simulink model "attitude_determination"  (R2024b)
settings: Solver=VariableStepAuto  StartTime=0.0  StopTime=inf  RelTol=1e-3
libraries: simulink x1
settings Model: Creator=boude  LastModifiedBy=boude

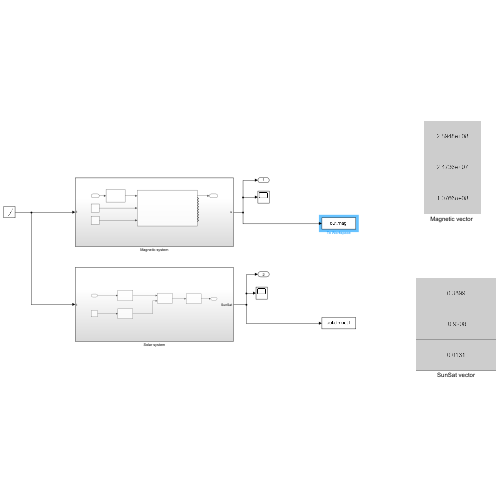
[thumbnail: Simulink's stored preview of the top-level diagram]
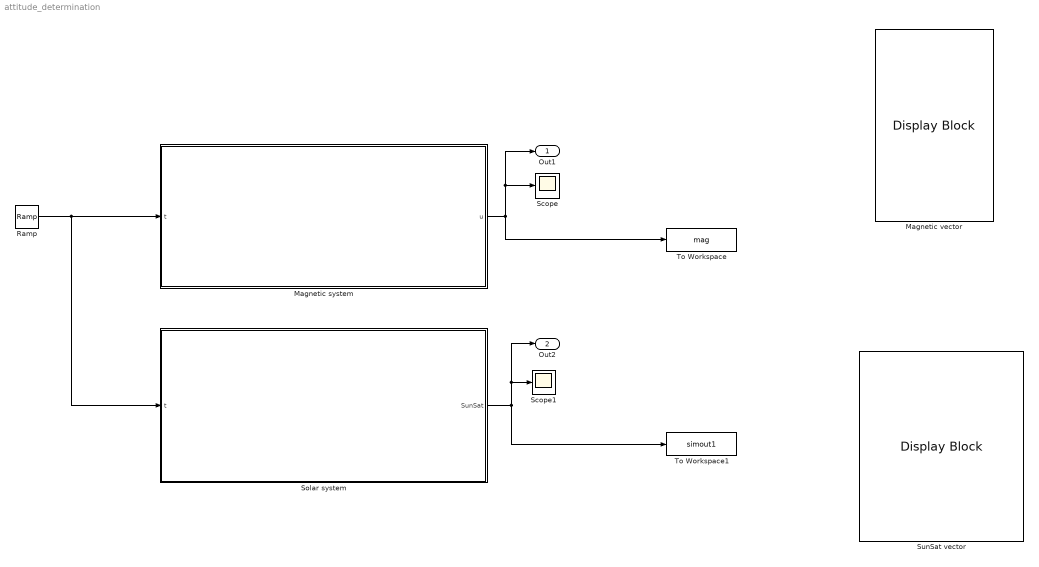
== system attitude_determination ==
  Magnetic system : Subsystem
  "Magnetic vector " : DisplayBlock  LabelPosition=Hide  Transparency=1  Layout=Fill available space
  Ramp : simulink/Sources/Ramp  slope=1  start=1  InitialOutput=1
  Scope : Scope
  Scope1 : Scope
  Solar system : Subsystem
  SunSat vector : DisplayBlock  LabelPosition=Hide  Transparency=1
  To Workspace : ToWorkspace  VariableName=mag  SampleTime=-1
      settings: Save2DSignal=2-D array (concatenate along first dimension)
  To Workspace1 : ToWorkspace  VariableName=simout1  SaveFormat=Timeseries  SampleTime=-1
  Out1 : Outport
  Out2 : Outport  Port=2
  wires:
  Ramp/1 -> Solar system/1(t), Magnetic system/1(t)
  Magnetic system/1(u) -> To Workspace/1, Out1/1, Scope/1
  Solar system/1(SunSat) -> To Workspace1/1, Out2/1, Scope1/1

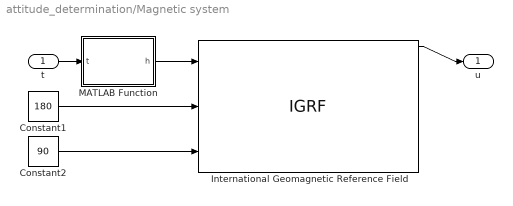
== system attitude_determination/Magnetic system ==
  t : Inport
  Constant1 : Constant  Value=180
  Constant2 : Constant  Value=90
  International Geomagnetic Reference Field : IGRF  units=English  time_in=off  month=December  day=6  year=2003
      settings: AttributesFormatString=%<generation>
  MATLAB Function : MATLAB Function  TreatAsAtomicUnit=on
  u : Outport
  wires:
  International Geomagnetic Reference Field/1 -> u/1
  Constant2/1 -> International Geomagnetic Reference Field/3
  Constant1/1 -> International Geomagnetic Reference Field/2
  MATLAB Function/1(h) -> International Geomagnetic Reference Field/1
  t/1 -> MATLAB Function/1(t)

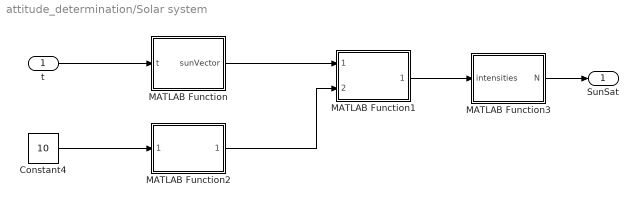
== system attitude_determination/Solar system ==
  t : Inport
  Constant4 : Constant  Value=10
  MATLAB Function : MATLAB Function  TreatAsAtomicUnit=on
  MATLAB Function1 : MATLAB Function  TreatAsAtomicUnit=on
  MATLAB Function2 : MATLAB Function  TreatAsAtomicUnit=on
  MATLAB Function3 : MATLAB Function  TreatAsAtomicUnit=on
  SunSat : Outport
  wires:
  Constant4/1 -> MATLAB Function2/1(omega)
  MATLAB Function/1(sunVector) -> MATLAB Function1/1(sunVec)
  MATLAB Function2/1(R_cubesat) -> MATLAB Function1/2(R_cubesat)
  t/1 -> MATLAB Function/1(t)
  MATLAB Function1/1(intensities) -> MATLAB Function3/1(intensities)
  MATLAB Function3/1(N) -> SunSat/1

== matlab function attitude_determination/Solar system/MATLAB Function ==
  data: t input; sunVector output
function sunVector  = sunPositionSimple(t)
% sunPositionSimple : calcul approximatif du vecteur unitaire pointant vers le Soleil
% Inputs:
%   - dayOfYear : jour de l'année (1 à 365)
%   - timeUTC : heure en décimal UTC (ex: 13.5 = 13h30 UTC)
% Output:
%   - sunVector : vecteur 3D unitaire [x;y;z] pointant vers le soleil en coordonnées ENU (Est-Nord-Haut)
    dayOfYear = floor(t / 86400) + 1;
    timeUTC = mod(t, 86400) / 3600;  % heure en décimal

    % Constantes
    lat = 48.8566;    % latitude Paris (°)
    lon = 2.3522;     % longitude Paris (°)
    
    % Calcul de l'angle horaire solaire (en degrés)
    % On suppose que midi solaire correspond à 12h heure locale
    % Correction décalage longitude vers UTC
    localTime = timeUTC + lon/15; % Convertit UTC en heure solaire approximative locale
    
    % Angle horaire solaire (omega) en degrés, midi solaire = 0°, matin négatif, après-midi positif
    omega = 15 * (localTime - 12);
    
    % Déclinaison solaire approximative (en degrés)
    % Approximation simple en fonction du jour de l'année (formule trigonométrique)
    declin = 23.44 * sind(360 * (284 + dayOfYear) / 365);
    
    % Calcul de l'angle zénithal solaire (theta_sun)
    cos_theta = sind(lat) * sind(declin) + cosd(lat) * cosd(declin) * cosd(omega);
    theta_sun = acosd(cos_theta);  % en degrés
    
    % Calcul de l'azimut solaire (phi_sun) approximatif (degrés, depuis le sud, vers l'ouest)
    sin_phi = -(cosd(declin) * sind(omega)) / sind(theta_sun);
    cos_phi = (sind(declin) - sind(lat) * cosd(theta_sun)) / (cosd(lat) * sind(theta_sun));
    phi_sun = atan2d(sin_phi, cos_phi);
    
    % Passage à un vecteur unitaire (système de coordonnées ENU)
    % x = Est, y = Nord, z = Haut
    % Azimut depuis le sud vers l'ouest → on recentre vers Est = 0°, Nord = 90°
    azimuth = mod(180 - phi_sun, 360); % azimut en degrés, 0 = Est, 90 = Nord
    
    % Convertir en radians
    zenith_rad = deg2rad(theta_sun);
    azimuth_rad = deg2rad(azimuth);
    
    % Composantes cartésiennes
    x = sin(zenith_rad) * cos(azimuth_rad);
    y = sin(zenith_rad) * sin(azimuth_rad);
    z = cos(zenith_rad);
    
    sunVector = [x; y; z];

    if theta_sun > 90
        sunVector = [0; 0; 0];
    end
    
end

== matlab function attitude_determination/Solar system/MATLAB Function2 ==
  data: omega input; R_cubesat output
function R_cubesat = fcn(omega)
t = 60;
theta = deg2rad(omega * t); % omega in deg/s, t in seconds
R_cubesat = [cos(theta), -sin(theta), 0;
     sin(theta),  cos(theta), 0;
     0,           0,          1];

== matlab function attitude_determination/Magnetic system/MATLAB Function ==
  data: h output; t input
function h = altitudeVariation(t)
% altitudeVariation : donne l'altitude en fonction du temps t (en secondes)
% h(t) = 500 + 100 * sin(2π * t / 600)

    h = 500 + 100 * sin(2 * pi * t / 600);
end

== matlab function attitude_determination/Solar system/MATLAB Function3 ==
  data: intensities input; N output
function N = sunSatelliteVector(intensities)
% sunSatelliteVector : calcule le vecteur Soleil-Satellite à partir des intensités mesurées
% Input:
%   - intensities : [6x1] vecteur contenant l’intensité sur chaque panneau solaire
% Output:
%   - N : [3x1] vecteur unitaire directionnel Soleil-Satellite

    % Normales des 6 faces du CubeSat (X+, X-, Y+, Y-, Z+, Z-)
    normals = [ 1  0  0;   % Face X+
               -1  0  0;   % Face X-
                0  1  0;   % Face Y+
                0 -1  0;   % Face Y-
                0  0  1;   % Face Z+
                0  0 -1];  % Face Z-

    % Numérateur : somme pondérée des normales
    numerator = zeros(1,3);
    for i = 1:6
        numerator = numerator + intensities(i) * normals(i,:);
    end

    % Dénominateur : somme des intensités
    denominator = sum(intensities);

    % Si toutes les intensités sont nulles → soleil non visible
    if denominator < 1e-3  % seuil de sécurité
        N = [0; 0; 0];  % ou NaN(3,1) si tu veux signaler l'absence de lumière
        return;
    end

    % Calcul du vecteur normalisé
    N = (numerator / denominator)';  % transpose pour avoir un vecteur colonne
    N = N / norm(N);  % normalisation finale
end

== matlab function attitude_determination/Solar system/MATLAB Function1 ==
  data: sunVec input; intensities output; R_cubesat input
function intensities = SolarPanelsResponse(sunVec, R_cubesat)
% sunVec : [3x1] vecteur Soleil (dans le repère inertiel ou local)
% R_cubesat : [3x3] matrice de rotation (orientation du CubeSat)
% intensities : [6x1] intensité sur chaque panneau

% Normaliser le vecteur Soleil
sunVec = sunVec / norm(sunVec);

% Exprimer le vecteur Soleil dans le repère du CubeSat
sunVec_body = R_cubesat * sunVec;

% Normales des 6 faces (X+, X−, Y+, Y−, Z+, Z−)
normals = [ 1  0  0;   % Face X+
           -1  0  0;   % Face X-
            0  1  0;   % Face Y+
            0 -1  0;   % Face Y-
            0  0  1;   % Face Z+
            0  0 -1];  % Face Z-

% Calcul de l’intensité reçue sur chaque face
intensities = max(0,normals * sunVec_body) ; % 6x1
